simulink model "PID_Controller2_crazyfliemodel"  (R2016b)
settings: Solver=ode4  StartTime=0.0  StopTime=50  FixedStep=.01  RelTol=1e-5
InitFcn:
  | parameters;
values from neighbouring files (symbols this model uses):
  pwm = (we-4070.3)/0.2685    [parameters.m]
undefined symbols (not defined in the file or in its folder): delay1, quad
(part 1 of 2)
settings Model: Creator=corkep  LastModifiedBy=fmobini
settings SolverCC: AlgebraicLoopSolver=LineSearch
settings DataIOCC: LimitDataPoints=on  SaveFormat=Array  SignalLoggingSaveFormat=ModelDataLogs
settings OptimizationCC: BlockReduction=off  BooleanDataType=off  LifeSpan=inf
settings DebuggingCC: SaveWithParameterizedLinksMsg=none  UnderspecifiedInitializationDetection=Classic  MergeDetectMultiDrivingBlocksExec=none  SignalResolutionControl=TryResolveAllWithWarning  MultiTaskDSMMsg=warning  MultiTaskCondExecSysMsg=none  AllowSymbolicDim=off  StateNameClashWarn=warning  SFUnexpectedBacktrackingDiag=warning  SFNoUnconditionalDefaultTransitionDiag=warning  SFExecutionAtInitializationDiag=none
settings HardwareCC: ProdBitPerPointer=32  ProdBitPerSizeT=32  ProdBitPerPtrDiffT=32  ProdLargestAtomicFloat=None  ProdIntDivRoundTo=Undefined  ProdEndianess=Unspecified  ProdWordSize=32  ProdHWDeviceType=32-bit Generic  TargetBitPerPointer=64  TargetBitPerSizeT=64  TargetBitPerPtrDiffT=64  TargetLongLongMode=on  TargetIntDivRoundTo=Zero  TargetEndianess=LittleEndian  TargetWordSize=64  TargetHWDeviceType=MATLAB Host  ProdEqTarget=off
settings ModelReferenceCC: PropagateSignalLabelsOutOfModel=off
settings GRTTargetCC: TargetLangStandard=C89/C90 (ANSI)  GeneratePreprocessorConditionals=Disable all
settings ConfigComp: CovMetricSettings=dw  CovHtmlReporting=on  CovSaveCumulativeToWorkspaceVar=on  CovSaveSingleToWorkspaceVar=on  CovExternalEMLEnable=off

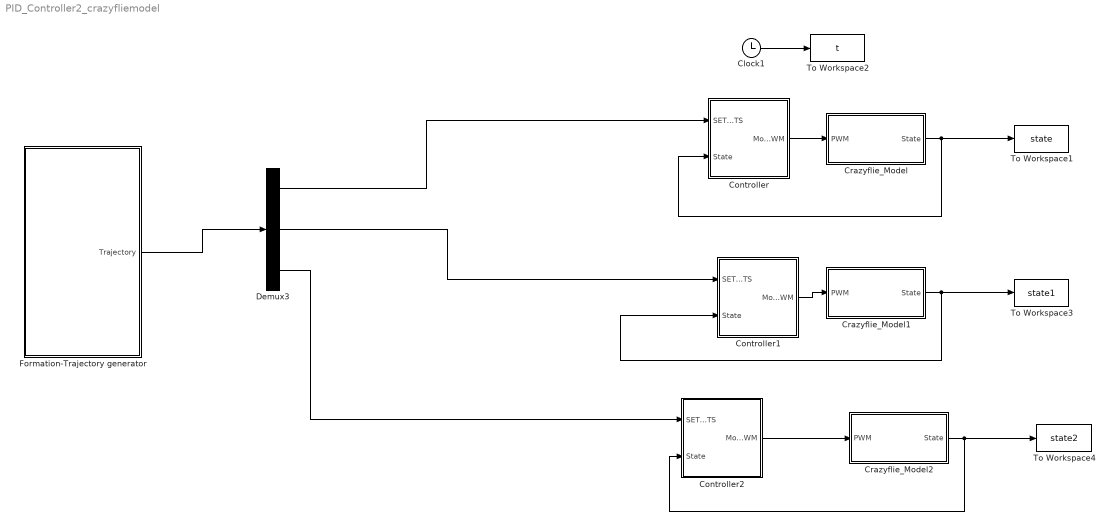
== system PID_Controller2_crazyfliemodel ==
  " Formation-Trajectory generator" : Subsystem
  Clock1 : Clock
  Controller : Subsystem  TreatAsAtomicUnit=on
  Controller1 : Subsystem  TreatAsAtomicUnit=on
  Controller2 : Subsystem  TreatAsAtomicUnit=on
  Crazyflie_Model : Subsystem
  Crazyflie_Model1 : Subsystem
  Crazyflie_Model2 : Subsystem
  Demux3 : Demux  Outputs=3
  To Workspace1 : ToWorkspace  VariableName=state  SampleTime=-1
  To Workspace2 : ToWorkspace  VariableName=t  SampleTime=-1
  To Workspace3 : ToWorkspace  VariableName=state1  SampleTime=-1
  To Workspace4 : ToWorkspace  VariableName=state2  SampleTime=-1
  wires:
  Clock1/1 -> To Workspace2/1
  Crazyflie_Model/1(State) -> To Workspace1/1, Controller/2(State)
  Controller/1(Motors_PWM) -> Crazyflie_Model/1(PWM)
  " Formation-Trajectory generator"/1(Trajectory) -> Demux3/1
  Demux3/1 -> Controller/1(SET-POINTS)
  Crazyflie_Model1/1(State) -> To Workspace3/1, Controller1/2(State)
  Controller1/1(Motors_PWM) -> Crazyflie_Model1/1(PWM)
  Demux3/2 -> Controller1/1(SET-POINTS)
  Crazyflie_Model2/1(State) -> To Workspace4/1, Controller2/2(State)
  Controller2/1(Motors_PWM) -> Crazyflie_Model2/1(PWM)
  Demux3/3 -> Controller2/1(SET-POINTS)

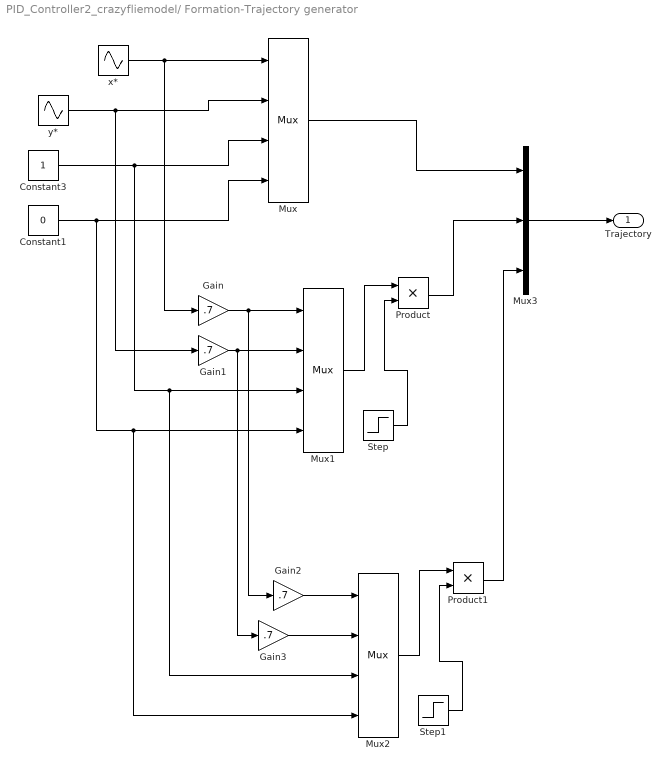
== system PID_Controller2_crazyfliemodel/ Formation-Trajectory generator ==
  Constant1 : Constant  Value=0
  Constant3 : Constant
  Gain{,1..3} (4 alike) : Gain  Gain=.7
  Mux : Mux
  Mux1 : Mux
  Mux2 : Mux
  Mux3 : Mux  Inputs=3
  Product : Product
  Product1 : Product
  Step : Step  Time=6  SampleTime=0
  Step1 : Step  Time=15  SampleTime=0
  x* : Sin  Amplitude=3  Frequency=2*pi*0.085
  y* : Sin  Amplitude=3  Frequency=2*pi*0.085  Phase=pi/2
  Trajectory : Outport
  wires:
  Constant3/1 -> Mux2/3, Mux1/3, Mux/3
  Constant1/1 -> Mux2/4, Mux1/4, Mux/4
  x*/1 -> Gain/1, Mux/1
  y*/1 -> Gain1/1, Mux/2
  Mux/1 -> Mux3/1
  Mux3/1 -> Trajectory/1
  Gain1/1 -> Gain3/1, Mux1/2
  Gain/1 -> Gain2/1, Mux1/1
  Gain2/1 -> Mux2/1
  Gain3/1 -> Mux2/2
  Product/1 -> Mux3/2
  Mux1/1 -> Product/1
  Step/1 -> Product/2
  Mux2/1 -> Product1/1
  Step1/1 -> Product1/2
  Product1/1 -> Mux3/3

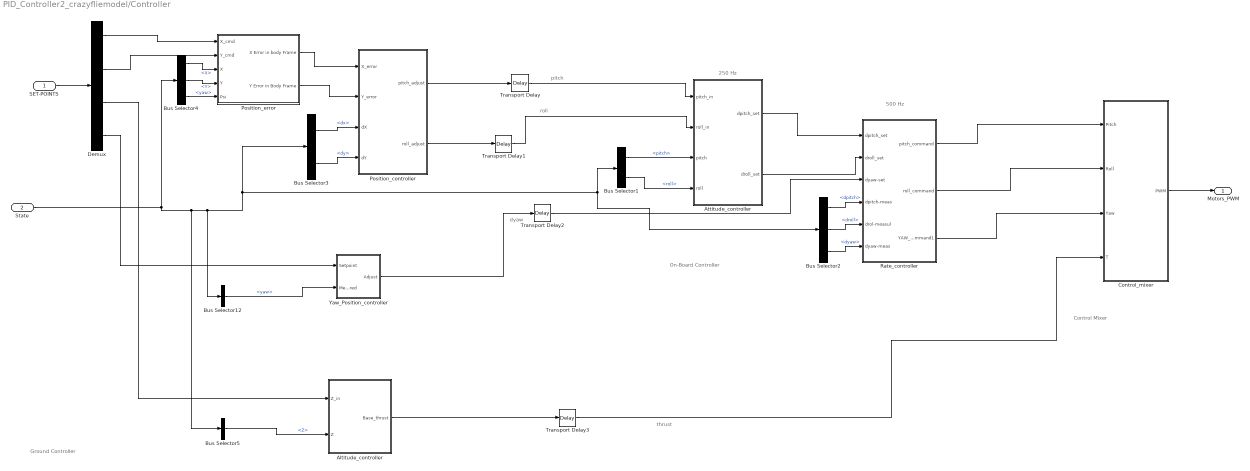
== system PID_Controller2_crazyfliemodel/Controller ==
  note: pitch
  note: Control Mixer
  note: On-Board Controller
  note: Ground Controller
  note: 250 Hz
  note: 500 Hz
  note: roll
  note: thrust
  note: dyaw
  SET-POINTS : Inport
  State : Inport  Port=2
  Altitude_controller : Subsystem
  Attitude_controller : Subsystem
  Bus Selector1 : BusSelector  OutputSignals=pitch,roll
  Bus Selector12 : BusSelector  OutputSignals=yaw
  Bus Selector2 : BusSelector  OutputSignals=dpitch,droll,dyaw
  Bus Selector3 : BusSelector  OutputSignals=dx,dy
  Bus Selector4 : BusSelector  OutputSignals=X,Y,yaw
  Bus Selector5 : BusSelector  OutputSignals=Z
  Control_mixer : Subsystem
  Demux : Demux
  Position_controller : Subsystem
  Position_error : Subsystem
  Rate_controller : Subsystem
  Transport Delay{,1..3} (4 alike) : TransportDelay  DelayTime=delay1
  Yaw_Position_controller : Subsystem
  Motors_PWM : Outport
  wires:
  Rate_controller/1(pitch_command) -> Control_mixer/1(Pitch)
  Rate_controller/2(roll_command) -> Control_mixer/2("Roll\t")
  Altitude_controller/1(Base_thrust) -> Transport Delay3/1
  Demux/3 -> Altitude_controller/1(Z_in)
  Bus Selector5/1 -> Altitude_controller/2(Z)  "<Z>"
  State/1 -> Bus Selector5/1, Bus Selector12/1, Bus Selector3/1, Bus Selector2/1, Bus Selector1/1, Bus Selector4/1
  Attitude_controller/1(dpitch_set) -> Rate_controller/1(dpitch_set)
  Attitude_controller/2(droll_set) -> Rate_controller/2(droll_set)
  Position_error/1(X Error in body Frame) -> Position_controller/1(X_error)
  Position_error/2(Y Error in Body Frame) -> Position_controller/2(Y_error)
  Position_controller/1(pitch_adjust) -> Transport Delay/1
  Bus Selector12/1 -> Yaw_Position_controller/2(Measured)  "<yaw>"
  Position_controller/2(roll_adjust) -> Transport Delay1/1
  Demux/1 -> Position_error/1(X_cmd)
  Demux/4 -> Yaw_Position_controller/1(Setpoint)
  Demux/2 -> Position_error/2(Y_cmd)
  SET-POINTS/1 -> Demux/1
  Yaw_Position_controller/1(Adjust) -> Transport Delay2/1
  Rate_controller/3(YAW_command1) -> Control_mixer/3(Yaw)
  Bus Selector1/1 -> Attitude_controller/3(pitch)  "<pitch>"
  Bus Selector1/2 -> Attitude_controller/4(roll)  "<roll>"
  Bus Selector2/1 -> Rate_controller/4(dpitch-meas)  "<dpitch>"
  Bus Selector2/2 -> Rate_controller/5(drol-measul)  "<droll>"
  Bus Selector2/3 -> Rate_controller/6(dyaw-meas)  "<dyaw>"
  Bus Selector3/1 -> Position_controller/3(dX)  "<dx>"
  Bus Selector3/2 -> Position_controller/4(dY)  "<dy>"
  Bus Selector4/1 -> Position_error/3(X)  "<X>"
  Bus Selector4/2 -> Position_error/4(Y)  "<Y>"
  Bus Selector4/3 -> Position_error/5(Psi)  "<yaw>"
  Control_mixer/1(PWM) -> Motors_PWM/1
  Transport Delay/1 -> Attitude_controller/1(pitch_in)
  Transport Delay1/1 -> Attitude_controller/2(roll_in)
  Transport Delay2/1 -> Rate_controller/3(dyaw-set)
  Transport Delay3/1 -> Control_mixer/4(T)

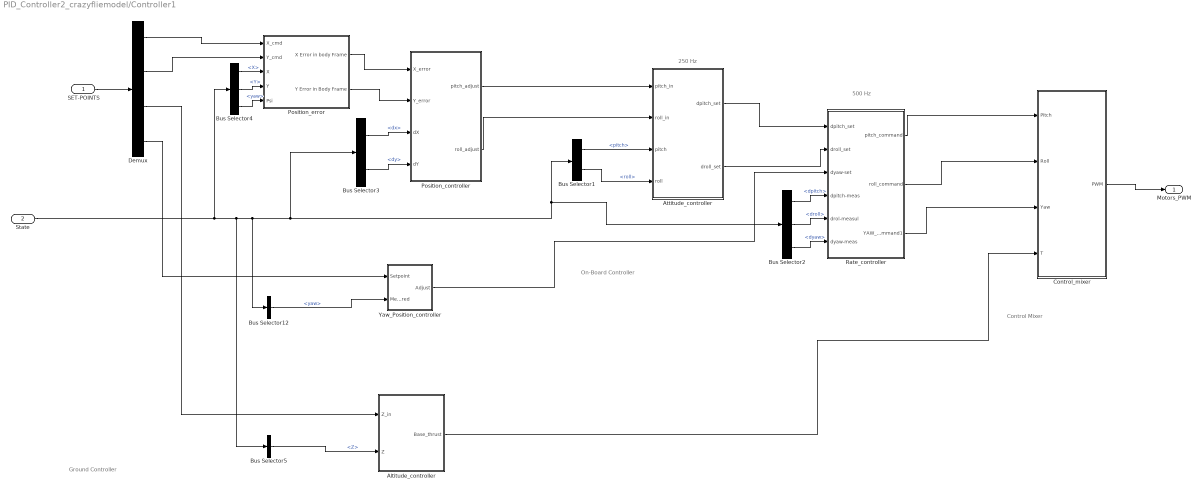
== system PID_Controller2_crazyfliemodel/Controller1 ==
  note: Control Mixer
  note: On-Board Controller
  note: Ground Controller
  note: 250 Hz
  note: 500 Hz
  SET-POINTS : Inport
  State : Inport  Port=2
  Altitude_controller : Subsystem
  Attitude_controller : Subsystem
  Bus Selector1 : BusSelector  OutputSignals=pitch,roll
  Bus Selector12 : BusSelector  OutputSignals=yaw
  Bus Selector2 : BusSelector  OutputSignals=dpitch,droll,dyaw
  Bus Selector3 : BusSelector  OutputSignals=dx,dy
  Bus Selector4 : BusSelector  OutputSignals=X,Y,yaw
  Bus Selector5 : BusSelector  OutputSignals=Z
  Control_mixer : Subsystem
  Demux : Demux
  Position_controller : Subsystem
  Position_error : Subsystem
  Rate_controller : Subsystem
  Yaw_Position_controller : Subsystem
  Motors_PWM : Outport
  wires:
  Control_mixer/1(PWM) -> Motors_PWM/1
  Rate_controller/1(pitch_command) -> Control_mixer/1(Pitch)
  Rate_controller/2(roll_command) -> Control_mixer/2("Roll\t")
  Altitude_controller/1(Base_thrust) -> Control_mixer/4(T)
  Demux/3 -> Altitude_controller/1(Z_in)
  Bus Selector5/1 -> Altitude_controller/2(Z)  "<Z>"
  State/1 -> Bus Selector4/1, Bus Selector5/1, Bus Selector12/1, Bus Selector3/1, Bus Selector2/1, Bus Selector1/1
  Attitude_controller/1(dpitch_set) -> Rate_controller/1(dpitch_set)
  Attitude_controller/2(droll_set) -> Rate_controller/2(droll_set)
  Position_error/1(X Error in body Frame) -> Position_controller/1(X_error)
  Position_error/2(Y Error in Body Frame) -> Position_controller/2(Y_error)
  Position_controller/1(pitch_adjust) -> Attitude_controller/1(pitch_in)
  Bus Selector12/1 -> Yaw_Position_controller/2(Measured)  "<yaw>"
  Position_controller/2(roll_adjust) -> Attitude_controller/2(roll_in)
  Demux/1 -> Position_error/1(X_cmd)
  Demux/4 -> Yaw_Position_controller/1(Setpoint)
  Demux/2 -> Position_error/2(Y_cmd)
  SET-POINTS/1 -> Demux/1
  Yaw_Position_controller/1(Adjust) -> Rate_controller/3(dyaw-set)
  Rate_controller/3(YAW_command1) -> Control_mixer/3(Yaw)
  Bus Selector1/1 -> Attitude_controller/3(pitch)  "<pitch>"
  Bus Selector1/2 -> Attitude_controller/4(roll)  "<roll>"
  Bus Selector2/1 -> Rate_controller/4(dpitch-meas)  "<dpitch>"
  Bus Selector2/2 -> Rate_controller/5(drol-measul)  "<droll>"
  Bus Selector2/3 -> Rate_controller/6(dyaw-meas)  "<dyaw>"
  Bus Selector3/1 -> Position_controller/3(dX)  "<dx>"
  Bus Selector3/2 -> Position_controller/4(dY)  "<dy>"
  Bus Selector4/1 -> Position_error/3(X)  "<X>"
  Bus Selector4/2 -> Position_error/4(Y)  "<Y>"
  Bus Selector4/3 -> Position_error/5(Psi)  "<yaw>"

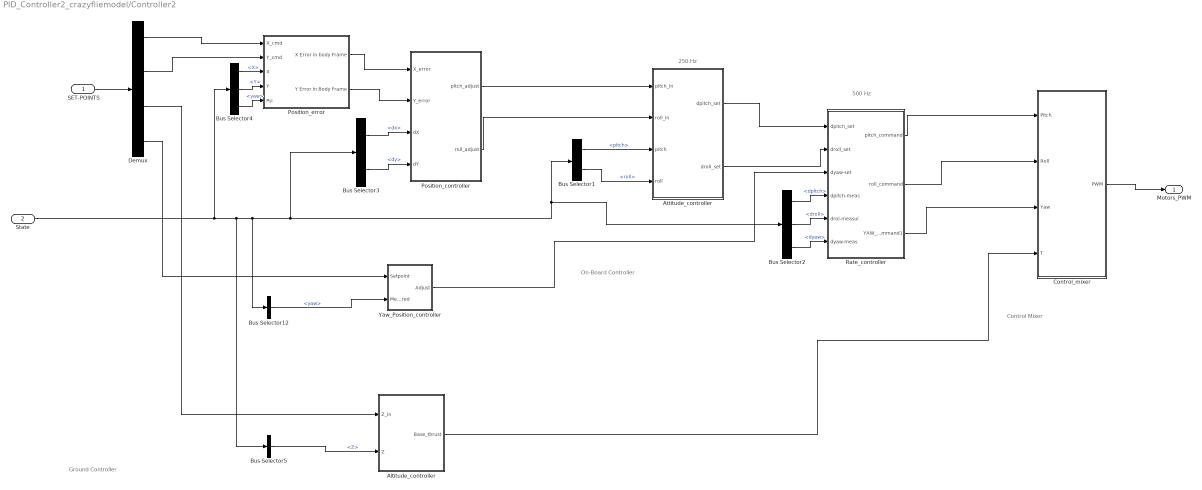
== system PID_Controller2_crazyfliemodel/Controller2 ==
  note: Control Mixer
  note: On-Board Controller
  note: Ground Controller
  note: 250 Hz
  note: 500 Hz
  SET-POINTS : Inport
  State : Inport  Port=2
  Altitude_controller : Subsystem
  Attitude_controller : Subsystem
  Bus Selector1 : BusSelector  OutputSignals=pitch,roll
  Bus Selector12 : BusSelector  OutputSignals=yaw
  Bus Selector2 : BusSelector  OutputSignals=dpitch,droll,dyaw
  Bus Selector3 : BusSelector  OutputSignals=dx,dy
  Bus Selector4 : BusSelector  OutputSignals=X,Y,yaw
  Bus Selector5 : BusSelector  OutputSignals=Z
  Control_mixer : Subsystem
  Demux : Demux
  Position_controller : Subsystem
  Position_error : Subsystem
  Rate_controller : Subsystem
  Yaw_Position_controller : Subsystem
  Motors_PWM : Outport
  wires:
  Control_mixer/1(PWM) -> Motors_PWM/1
  Rate_controller/1(pitch_command) -> Control_mixer/1(Pitch)
  Rate_controller/2(roll_command) -> Control_mixer/2("Roll\t")
  Altitude_controller/1(Base_thrust) -> Control_mixer/4(T)
  Demux/3 -> Altitude_controller/1(Z_in)
  Bus Selector5/1 -> Altitude_controller/2(Z)  "<Z>"
  State/1 -> Bus Selector4/1, Bus Selector5/1, Bus Selector12/1, Bus Selector3/1, Bus Selector2/1, Bus Selector1/1
  Attitude_controller/1(dpitch_set) -> Rate_controller/1(dpitch_set)
  Attitude_controller/2(droll_set) -> Rate_controller/2(droll_set)
  Position_error/1(X Error in body Frame) -> Position_controller/1(X_error)
  Position_error/2(Y Error in Body Frame) -> Position_controller/2(Y_error)
  Position_controller/1(pitch_adjust) -> Attitude_controller/1(pitch_in)
  Bus Selector12/1 -> Yaw_Position_controller/2(Measured)  "<yaw>"
  Position_controller/2(roll_adjust) -> Attitude_controller/2(roll_in)
  Demux/1 -> Position_error/1(X_cmd)
  Demux/4 -> Yaw_Position_controller/1(Setpoint)
  Demux/2 -> Position_error/2(Y_cmd)
  SET-POINTS/1 -> Demux/1
  Yaw_Position_controller/1(Adjust) -> Rate_controller/3(dyaw-set)
  Rate_controller/3(YAW_command1) -> Control_mixer/3(Yaw)
  Bus Selector1/1 -> Attitude_controller/3(pitch)  "<pitch>"
  Bus Selector1/2 -> Attitude_controller/4(roll)  "<roll>"
  Bus Selector2/1 -> Rate_controller/4(dpitch-meas)  "<dpitch>"
  Bus Selector2/2 -> Rate_controller/5(drol-measul)  "<droll>"
  Bus Selector2/3 -> Rate_controller/6(dyaw-meas)  "<dyaw>"
  Bus Selector3/1 -> Position_controller/3(dX)  "<dx>"
  Bus Selector3/2 -> Position_controller/4(dY)  "<dy>"
  Bus Selector4/1 -> Position_error/3(X)  "<X>"
  Bus Selector4/2 -> Position_error/4(Y)  "<Y>"
  Bus Selector4/3 -> Position_error/5(Psi)  "<yaw>"

== system PID_Controller2_crazyfliemodel/Crazyflie_Model ==
  PWM : Inport
  DYNAMICS MODEL : Subsystem
  Motor MODEL : Subsystem
  State : Outport
  wires:
  PWM/1 -> Motor MODEL/1(PWM)
  Motor MODEL/1(Thrust) -> DYNAMICS MODEL/1(THRUST)
  Motor MODEL/2(Moment) -> DYNAMICS MODEL/2(MOMENT)
  DYNAMICS MODEL/1(STATES) -> State/1

== system PID_Controller2_crazyfliemodel/Crazyflie_Model1 ==
  PWM : Inport
  DYNAMICS MODEL : Subsystem
  Motor MODEL : Subsystem
  State : Outport
  wires:
  PWM/1 -> Motor MODEL/1(PWM)
  Motor MODEL/1(Thrust) -> DYNAMICS MODEL/1(THRUST)
  Motor MODEL/2(Moment) -> DYNAMICS MODEL/2(MOMENT)
  DYNAMICS MODEL/1(STATES) -> State/1

== system PID_Controller2_crazyfliemodel/Crazyflie_Model2 ==
  PWM : Inport
  DYNAMICS MODEL : Subsystem
  Motor MODEL : Subsystem
  State : Outport
  wires:
  PWM/1 -> Motor MODEL/1(PWM)
  Motor MODEL/1(Thrust) -> DYNAMICS MODEL/1(THRUST)
  Motor MODEL/2(Moment) -> DYNAMICS MODEL/2(MOMENT)
  DYNAMICS MODEL/1(STATES) -> State/1

== system PID_Controller2_crazyfliemodel/Controller/Altitude_controller ==
  Z_in : Inport
  Z : Inport  Port=2
  "Min_thrust " : Constant  Value=pwm  SampleTime=0
  PID_Altitude : Subsystem
  Saturation : Saturate  UpperLimit=60000  LowerLimit=-20000
  Saturation1 : Saturate  UpperLimit=15000  LowerLimit=-20000
  Sum3 : Sum  Inputs=|++
  Base_thrust : Outport
  wires:
  Saturation/1 -> Base_thrust/1
  "Min_thrust "/1 -> Sum3/2
  Sum3/1 -> Saturation/1
  Z/1 -> PID_Altitude/2(Measured)
  Z_in/1 -> PID_Altitude/1(Setpoint)
  Saturation1/1 -> Sum3/1
  PID_Altitude/1(Adjust) -> Saturation1/1

== system PID_Controller2_crazyfliemodel/Controller/Attitude_controller ==
  pitch_in : Inport
  roll_in : Inport  Port=2
  pitch : Inport  Port=3
  roll : Inport  Port=4
  Gain1 : Gain  Gain=180/pi
  Gain3 : Gain  Gain=180/pi
  PID_pitch_Rate2 : Subsystem
  PID_roll_Rate1 : Subsystem
  dpitch_set : Outport
  droll_set : Outport  Port=2
  wires:
  roll_in/1 -> PID_roll_Rate1/1(Setpoint)
  roll/1 -> Gain1/1
  PID_roll_Rate1/1(Adjust) -> droll_set/1
  pitch_in/1 -> PID_pitch_Rate2/1(Setpoint)
  pitch/1 -> Gain3/1
  PID_pitch_Rate2/1(Adjust) -> dpitch_set/1
  Gain3/1 -> PID_pitch_Rate2/2(Measured)
  Gain1/1 -> PID_roll_Rate1/2(Measured)

== system PID_Controller2_crazyfliemodel/Controller/Control_mixer ==
  Pitch : Inport
  "Roll\t" : Inport  Port=2
  Yaw : Inport  Port=3
  T : Inport  Port=4
  Gain : Gain  Gain=0.5
  Gain1 : Gain  Gain=0.5
  Mux : Mux
  Sum1 : Sum  Inputs=|+-+  SaturateOnIntegerOverflow=on  InputSameDT=on  OutDataTypeStr=Inherit: Same as first input
  Sum{9..12} (4 alike) : Sum  Inputs=|++  SaturateOnIntegerOverflow=on  InputSameDT=on  OutDataTypeStr=Inherit: Same as first input
  Sum3 : Sum  Inputs=|++-  SaturateOnIntegerOverflow=on  InputSameDT=on  OutDataTypeStr=Inherit: Same as first input
  Sum5 : Sum  Inputs=|+-+  SaturateOnIntegerOverflow=on  InputSameDT=on  OutDataTypeStr=Inherit: Same as first input
  Sum7 : Sum  Inputs=|---  SaturateOnIntegerOverflow=on  InputSameDT=on  OutDataTypeStr=Inherit: Same as first input
  PWM : Outport
  wires:
  Sum3/1 -> Sum11/1
  Yaw/1 -> Sum5/3, Sum3/3, Sum7/3, Sum1/3
  T/1 -> Sum11/2, Sum12/2, Sum10/2, Sum9/2
  Sum5/1 -> Sum12/1
  Sum7/1 -> Sum9/1
  Sum1/1 -> Sum10/1
  "Roll\t"/1 -> Gain1/1
  Pitch/1 -> Gain/1
  Gain/1 -> Sum7/1, Sum1/1, Sum5/2, Sum3/2
  Gain1/1 -> Sum7/2, Sum1/2, Sum5/1, Sum3/1
  Sum9/1 -> Mux/1
  Sum10/1 -> Mux/2
  Sum11/1 -> Mux/3
  Sum12/1 -> Mux/4
  Mux/1 -> PWM/1

== system PID_Controller2_crazyfliemodel/Controller/Position_controller ==
  X_error : Inport
  Y_error : Inport  Port=2
  dX : Inport  Port=3
  dY : Inport  Port=4
  PID_pitch_Rate2 : Subsystem
  PID_roll_Rate3 : Subsystem
  Saturation : Saturate  UpperLimit=30  LowerLimit=-30
  Saturation1 : Saturate  UpperLimit=30  LowerLimit=-30
  Scope1 : Scope
  Scope2 : Scope
  pitch_adjust : Outport
  roll_adjust : Outport  Port=2
  wires:
  Saturation1/1 -> roll_adjust/1
  PID_roll_Rate3/1(Adjust) -> Saturation1/1
  Saturation/1 -> pitch_adjust/1, Scope1/1
  PID_pitch_Rate2/1(Adjust) -> Saturation/1, Scope2/1
  dX/1 -> PID_pitch_Rate2/2(Measured)
  X_error/1 -> PID_pitch_Rate2/1(Setpoint)
  dY/1 -> PID_roll_Rate3/2(Measured)
  Y_error/1 -> PID_roll_Rate3/1(Setpoint)

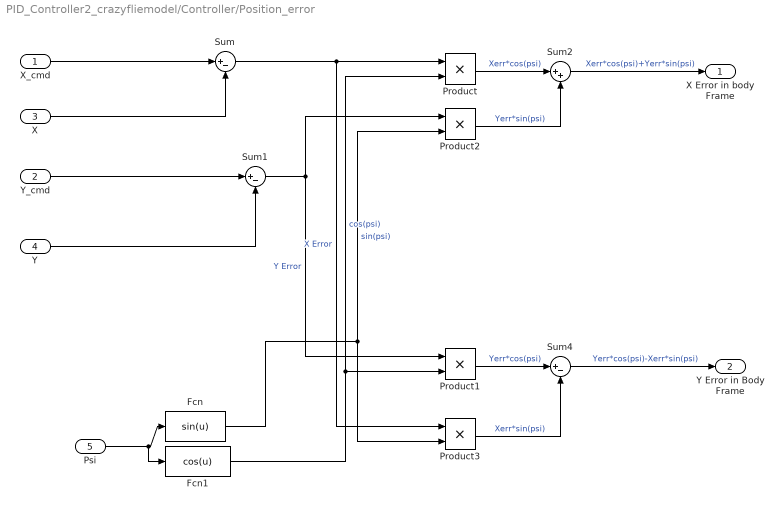
== system PID_Controller2_crazyfliemodel/Controller/Position_error ==
  X_cmd : Inport
  Y_cmd : Inport  Port=2
  X : Inport  Port=3
  Y : Inport  Port=4
  Psi : Inport  Port=5
  Fcn : Fcn  Expr=sin(u)
  Fcn1 : Fcn  Expr=cos(u)
  Product{,1..3} (4 alike) : Product
  Sum : Sum  Inputs=|+-
  Sum1 : Sum  Inputs=|+-
  Sum2 : Sum  Inputs=|++
  Sum4 : Sum  Inputs=|+-
  X Error in body Frame : Outport
  Y Error in Body Frame : Outport  Port=2
  wires:
  Sum4/1 -> Y Error in Body Frame/1  "Yerr*cos(psi)-Xerr*sin(psi)"
  Product3/1 -> Sum4/2  "Xerr*sin(psi)"
  Sum1/1 -> Product2/1, Product1/1  "Y Error"
  Fcn/1 -> Product3/2, Product2/2  "sin(psi)"
  Sum2/1 -> X Error in body Frame/1  "Xerr*cos(psi)+Yerr*sin(psi)"
  Y_cmd/1 -> Sum1/1
  X_cmd/1 -> Sum/1
  X/1 -> Sum/2
  Y/1 -> Sum1/2
  Sum/1 -> Product3/1, Product/1  "X Error"
  Fcn1/1 -> Product/2, Product1/2  "cos(psi)"
  Product/1 -> Sum2/1  "Xerr*cos(psi)"
  Product2/1 -> Sum2/2  "Yerr*sin(psi)"
  Product1/1 -> Sum4/1  "Yerr*cos(psi)"
  Psi/1 -> Fcn1/1, Fcn/1

== system PID_Controller2_crazyfliemodel/Controller/Rate_controller ==
  dpitch_set : Inport
  droll_set : Inport  Port=2
  dyaw-set : Inport  Port=3
  dpitch-meas : Inport  Port=4
  drol-measul : Inport  Port=5
  dyaw-meas : Inport  Port=6
  Gain1 : Gain  Gain=180/pi
  Gain4 : Gain  Gain=180/pi
  Gain7 : Gain  Gain=180/pi
  PID_Roll_Rate1 : Subsystem
  PID_Roll_Rate3 : Subsystem
  PID_YAW_Rate1 : Subsystem
  pitch_command : Outport
  roll_command : Outport  Port=2
  YAW_command1 : Outport  Port=3
  wires:
  dpitch_set/1 -> PID_Roll_Rate3/1(Setpoint)
  PID_Roll_Rate3/1(Adjust) -> pitch_command/1
  droll_set/1 -> PID_Roll_Rate1/1(Setpoint)
  drol-measul/1 -> Gain4/1
  PID_Roll_Rate1/1(Adjust) -> roll_command/1
  PID_YAW_Rate1/1(Adjust) -> YAW_command1/1
  dyaw-set/1 -> PID_YAW_Rate1/1(Setpoint)
  dyaw-meas/1 -> Gain7/1
  Gain7/1 -> PID_YAW_Rate1/2(Measured)
  Gain4/1 -> PID_Roll_Rate1/2(Measured)
  dpitch-meas/1 -> Gain1/1
  Gain1/1 -> PID_Roll_Rate3/2(Measured)

== system PID_Controller2_crazyfliemodel/Controller/Yaw_Position_controller ==
  Setpoint : Inport
  Measured : Inport  Port=2
  Gain6 : Gain  Gain=180/pi
  Kp : Gain  Gain=3  OutMin=[-200]  OutMax=[200]
  Saturation1 : Saturate  UpperLimit=200  LowerLimit=-200
  Sum6 : Sum  Inputs=+-|
  Adjust : Outport
  wires:
  Measured/1 -> Gain6/1  "measured"
  Setpoint/1 -> Sum6/1  "pid_desired"
  Kp/1 -> Saturation1/1
  Sum6/1 -> Kp/1  "pid_error"
  Gain6/1 -> Sum6/2
  Saturation1/1 -> Adjust/1

== system PID_Controller2_crazyfliemodel/Controller1/Altitude_controller ==
  Z_in : Inport
  Z : Inport  Port=2
  "Min_thrust " : Constant  Value=pwm  SampleTime=0
  PID_Altitude : Subsystem
  Saturation : Saturate  UpperLimit=60000  LowerLimit=-20000
  Saturation1 : Saturate  UpperLimit=15000  LowerLimit=-20000
  Sum3 : Sum  Inputs=|++
  Base_thrust : Outport
  wires:
  Saturation/1 -> Base_thrust/1
  "Min_thrust "/1 -> Sum3/2
  Sum3/1 -> Saturation/1
  Z/1 -> PID_Altitude/2(Measured)
  Z_in/1 -> PID_Altitude/1(Setpoint)
  Saturation1/1 -> Sum3/1
  PID_Altitude/1(Adjust) -> Saturation1/1

== system PID_Controller2_crazyfliemodel/Controller1/Attitude_controller ==
  pitch_in : Inport
  roll_in : Inport  Port=2
  pitch : Inport  Port=3
  roll : Inport  Port=4
  Gain1 : Gain  Gain=180/pi
  Gain3 : Gain  Gain=180/pi
  PID_Roll_Rate1 : Subsystem
  PID_Roll_Rate2 : Subsystem
  dpitch_set : Outport
  droll_set : Outport  Port=2
  wires:
  roll_in/1 -> PID_Roll_Rate1/1(Setpoint)
  roll/1 -> Gain1/1
  PID_Roll_Rate1/1(Adjust) -> droll_set/1
  pitch_in/1 -> PID_Roll_Rate2/1(Setpoint)
  pitch/1 -> Gain3/1
  PID_Roll_Rate2/1(Adjust) -> dpitch_set/1
  Gain3/1 -> PID_Roll_Rate2/2(Measured)
  Gain1/1 -> PID_Roll_Rate1/2(Measured)

== system PID_Controller2_crazyfliemodel/Controller1/Control_mixer ==
  Pitch : Inport
  "Roll\t" : Inport  Port=2
  Yaw : Inport  Port=3
  T : Inport  Port=4
  Configuration_X1 : Subsystem
  Mux1 : Mux
  PWM : Outport
  wires:
  Pitch/1 -> Configuration_X1/1(Pitch)
  Configuration_X1/3(W3) -> Mux1/3
  Configuration_X1/4(W4) -> Mux1/4
  T/1 -> Configuration_X1/4(Tau)
  Yaw/1 -> Configuration_X1/3(Yaw)
  "Roll\t"/1 -> Configuration_X1/2(Roll)
  Configuration_X1/2(W2) -> Mux1/2
  Configuration_X1/1(W1) -> Mux1/1
  Mux1/1 -> PWM/1

== system PID_Controller2_crazyfliemodel/Controller1/Position_controller ==
  X_error : Inport
  Y_error : Inport  Port=2
  dX : Inport  Port=3
  dY : Inport  Port=4
  PID_Roll_Rate2 : Subsystem
  PID_Roll_Rate3 : Subsystem
  PID_X2 : Subsystem
  PID_Y2 : Subsystem
  Saturation : Saturate  UpperLimit=30  LowerLimit=-30
  Saturation1 : Saturate  UpperLimit=30  LowerLimit=-30
  Scope1 : Scope
  Scope2 : Scope
  pitch_adjust : Outport
  roll_adjust : Outport  Port=2
  wires:
  Saturation1/1 -> roll_adjust/1
  PID_Roll_Rate3/1(Adjust) -> Saturation1/1
  Saturation/1 -> pitch_adjust/1, Scope1/1
  PID_Roll_Rate2/1(Adjust) -> Saturation/1, Scope2/1
  dX/1 -> PID_Roll_Rate2/2(Measured)
  X_error/1 -> PID_Roll_Rate2/1(Setpoint)
  dY/1 -> PID_Roll_Rate3/2(Measured)
  Y_error/1 -> PID_Roll_Rate3/1(Setpoint)

== system PID_Controller2_crazyfliemodel/Controller1/Position_error ==
  X_cmd : Inport
  Y_cmd : Inport  Port=2
  X : Inport  Port=3
  Y : Inport  Port=4
  Psi : Inport  Port=5
  Fcn : Fcn  Expr=sin(u)
  Fcn1 : Fcn  Expr=cos(u)
  Product{,1..3} (4 alike) : Product
  Sum : Sum  Inputs=|+-
  Sum1 : Sum  Inputs=|+-
  Sum2 : Sum  Inputs=|++
  Sum4 : Sum  Inputs=|+-
  X Error in body Frame : Outport
  Y Error in Body Frame : Outport  Port=2
  wires:
  Sum4/1 -> Y Error in Body Frame/1  "Yerr*cos(psi)-Xerr*sin(psi)"
  Product3/1 -> Sum4/2  "Xerr*sin(psi)"
  Sum1/1 -> Product2/1, Product1/1  "Y Error"
  Fcn/1 -> Product3/2, Product2/2  "sin(psi)"
  Sum2/1 -> X Error in body Frame/1  "Xerr*cos(psi)+Yerr*sin(psi)"
  Y_cmd/1 -> Sum1/1
  X_cmd/1 -> Sum/1
  X/1 -> Sum/2
  Y/1 -> Sum1/2
  Sum/1 -> Product3/1, Product/1  "X Error"
  Fcn1/1 -> Product/2, Product1/2  "cos(psi)"
  Product/1 -> Sum2/1  "Xerr*cos(psi)"
  Product2/1 -> Sum2/2  "Yerr*sin(psi)"
  Product1/1 -> Sum4/1  "Yerr*cos(psi)"
  Psi/1 -> Fcn1/1, Fcn/1

== system PID_Controller2_crazyfliemodel/Controller1/Rate_controller ==
  dpitch_set : Inport
  droll_set : Inport  Port=2
  dyaw-set : Inport  Port=3
  dpitch-meas : Inport  Port=4
  drol-measul : Inport  Port=5
  dyaw-meas : Inport  Port=6
  Gain1 : Gain  Gain=180/pi
  Gain4 : Gain  Gain=180/pi
  Gain7 : Gain  Gain=180/pi
  PID_Roll_Rate1 : Subsystem
  PID_Roll_Rate3 : Subsystem
  PID_YAW_Rate1 : Subsystem
  pitch_command : Outport
  roll_command : Outport  Port=2
  YAW_command1 : Outport  Port=3
  wires:
  dpitch_set/1 -> PID_Roll_Rate3/1(Setpoint)
  PID_Roll_Rate3/1(Adjust) -> pitch_command/1
  droll_set/1 -> PID_Roll_Rate1/1(Setpoint)
  drol-measul/1 -> Gain4/1
  PID_Roll_Rate1/1(Adjust) -> roll_command/1
  PID_YAW_Rate1/1(Adjust) -> YAW_command1/1
  dyaw-set/1 -> PID_YAW_Rate1/1(Setpoint)
  dyaw-meas/1 -> Gain7/1
  Gain7/1 -> PID_YAW_Rate1/2(Measured)
  Gain4/1 -> PID_Roll_Rate1/2(Measured)
  dpitch-meas/1 -> Gain1/1
  Gain1/1 -> PID_Roll_Rate3/2(Measured)

== system PID_Controller2_crazyfliemodel/Controller1/Yaw_Position_controller ==
  Setpoint : Inport
  Measured : Inport  Port=2
  Gain6 : Gain  Gain=180/pi
  Kp : Gain  Gain=3  OutMin=[-200]  OutMax=[200]
  Saturation1 : Saturate  UpperLimit=200  LowerLimit=-200
  Sum6 : Sum  Inputs=+-|
  Adjust : Outport
  wires:
  Measured/1 -> Gain6/1  "measured"
  Setpoint/1 -> Sum6/1  "pid_desired"
  Kp/1 -> Saturation1/1
  Sum6/1 -> Kp/1  "pid_error"
  Gain6/1 -> Sum6/2
  Saturation1/1 -> Adjust/1

== system PID_Controller2_crazyfliemodel/Controller2/Altitude_controller ==
  Z_in : Inport
  Z : Inport  Port=2
  "Min_thrust " : Constant  Value=pwm  SampleTime=0
  PID_Altitude : Subsystem
  Saturation : Saturate  UpperLimit=60000  LowerLimit=-20000
  Saturation1 : Saturate  UpperLimit=15000  LowerLimit=-20000
  Sum3 : Sum  Inputs=|++
  Base_thrust : Outport
  wires:
  Saturation/1 -> Base_thrust/1
  "Min_thrust "/1 -> Sum3/2
  Sum3/1 -> Saturation/1
  Z/1 -> PID_Altitude/2(Measured)
  Z_in/1 -> PID_Altitude/1(Setpoint)
  Saturation1/1 -> Sum3/1
  PID_Altitude/1(Adjust) -> Saturation1/1

== system PID_Controller2_crazyfliemodel/Controller2/Attitude_controller ==
  pitch_in : Inport
  roll_in : Inport  Port=2
  pitch : Inport  Port=3
  roll : Inport  Port=4
  Gain1 : Gain  Gain=180/pi
  Gain3 : Gain  Gain=180/pi
  PID_Roll_Rate1 : Subsystem
  PID_Roll_Rate2 : Subsystem
  dpitch_set : Outport
  droll_set : Outport  Port=2
  wires:
  roll_in/1 -> PID_Roll_Rate1/1(Setpoint)
  roll/1 -> Gain1/1
  PID_Roll_Rate1/1(Adjust) -> droll_set/1
  pitch_in/1 -> PID_Roll_Rate2/1(Setpoint)
  pitch/1 -> Gain3/1
  PID_Roll_Rate2/1(Adjust) -> dpitch_set/1
  Gain3/1 -> PID_Roll_Rate2/2(Measured)
  Gain1/1 -> PID_Roll_Rate1/2(Measured)

== system PID_Controller2_crazyfliemodel/Controller2/Control_mixer ==
  Pitch : Inport
  "Roll\t" : Inport  Port=2
  Yaw : Inport  Port=3
  T : Inport  Port=4
  Configuration_X1 : Subsystem
  Mux1 : Mux
  PWM : Outport
  wires:
  Pitch/1 -> Configuration_X1/1(Pitch)
  Configuration_X1/3(W3) -> Mux1/3
  Configuration_X1/4(W4) -> Mux1/4
  T/1 -> Configuration_X1/4(Tau)
  Yaw/1 -> Configuration_X1/3(Yaw)
  "Roll\t"/1 -> Configuration_X1/2(Roll)
  Configuration_X1/2(W2) -> Mux1/2
  Configuration_X1/1(W1) -> Mux1/1
  Mux1/1 -> PWM/1

== system PID_Controller2_crazyfliemodel/Controller2/Position_controller ==
  X_error : Inport
  Y_error : Inport  Port=2
  dX : Inport  Port=3
  dY : Inport  Port=4
  PID_Roll_Rate2 : Subsystem
  PID_Roll_Rate3 : Subsystem
  PID_X2 : Subsystem
  PID_Y2 : Subsystem
  Saturation : Saturate  UpperLimit=30  LowerLimit=-30
  Saturation1 : Saturate  UpperLimit=30  LowerLimit=-30
  Scope1 : Scope
  Scope2 : Scope
  pitch_adjust : Outport
  roll_adjust : Outport  Port=2
  wires:
  Saturation1/1 -> roll_adjust/1
  PID_Roll_Rate3/1(Adjust) -> Saturation1/1
  Saturation/1 -> pitch_adjust/1, Scope1/1
  PID_Roll_Rate2/1(Adjust) -> Saturation/1, Scope2/1
  dX/1 -> PID_Roll_Rate2/2(Measured)
  X_error/1 -> PID_Roll_Rate2/1(Setpoint)
  dY/1 -> PID_Roll_Rate3/2(Measured)
  Y_error/1 -> PID_Roll_Rate3/1(Setpoint)

== system PID_Controller2_crazyfliemodel/Controller2/Position_error ==
  X_cmd : Inport
  Y_cmd : Inport  Port=2
  X : Inport  Port=3
  Y : Inport  Port=4
  Psi : Inport  Port=5
  Fcn : Fcn  Expr=sin(u)
  Fcn1 : Fcn  Expr=cos(u)
  Product{,1..3} (4 alike) : Product
  Sum : Sum  Inputs=|+-
  Sum1 : Sum  Inputs=|+-
  Sum2 : Sum  Inputs=|++
  Sum4 : Sum  Inputs=|+-
  X Error in body Frame : Outport
  Y Error in Body Frame : Outport  Port=2
  wires:
  Sum4/1 -> Y Error in Body Frame/1  "Yerr*cos(psi)-Xerr*sin(psi)"
  Product3/1 -> Sum4/2  "Xerr*sin(psi)"
  Sum1/1 -> Product2/1, Product1/1  "Y Error"
  Fcn/1 -> Product3/2, Product2/2  "sin(psi)"
  Sum2/1 -> X Error in body Frame/1  "Xerr*cos(psi)+Yerr*sin(psi)"
  Y_cmd/1 -> Sum1/1
  X_cmd/1 -> Sum/1
  X/1 -> Sum/2
  Y/1 -> Sum1/2
  Sum/1 -> Product3/1, Product/1  "X Error"
  Fcn1/1 -> Product/2, Product1/2  "cos(psi)"
  Product/1 -> Sum2/1  "Xerr*cos(psi)"
  Product2/1 -> Sum2/2  "Yerr*sin(psi)"
  Product1/1 -> Sum4/1  "Yerr*cos(psi)"
  Psi/1 -> Fcn1/1, Fcn/1

== system PID_Controller2_crazyfliemodel/Controller2/Rate_controller ==
  dpitch_set : Inport
  droll_set : Inport  Port=2
  dyaw-set : Inport  Port=3
  dpitch-meas : Inport  Port=4
  drol-measul : Inport  Port=5
  dyaw-meas : Inport  Port=6
  Gain1 : Gain  Gain=180/pi
  Gain4 : Gain  Gain=180/pi
  Gain7 : Gain  Gain=180/pi
  PID_Roll_Rate1 : Subsystem
  PID_Roll_Rate3 : Subsystem
  PID_YAW_Rate1 : Subsystem
  pitch_command : Outport
  roll_command : Outport  Port=2
  YAW_command1 : Outport  Port=3
  wires:
  dpitch_set/1 -> PID_Roll_Rate3/1(Setpoint)
  PID_Roll_Rate3/1(Adjust) -> pitch_command/1
  droll_set/1 -> PID_Roll_Rate1/1(Setpoint)
  drol-measul/1 -> Gain4/1
  PID_Roll_Rate1/1(Adjust) -> roll_command/1
  PID_YAW_Rate1/1(Adjust) -> YAW_command1/1
  dyaw-set/1 -> PID_YAW_Rate1/1(Setpoint)
  dyaw-meas/1 -> Gain7/1
  Gain7/1 -> PID_YAW_Rate1/2(Measured)
  Gain4/1 -> PID_Roll_Rate1/2(Measured)
  dpitch-meas/1 -> Gain1/1
  Gain1/1 -> PID_Roll_Rate3/2(Measured)

== system PID_Controller2_crazyfliemodel/Controller2/Yaw_Position_controller ==
  Setpoint : Inport
  Measured : Inport  Port=2
  Gain6 : Gain  Gain=180/pi
  Kp : Gain  Gain=3  OutMin=[-200]  OutMax=[200]
  Saturation1 : Saturate  UpperLimit=200  LowerLimit=-200
  Sum6 : Sum  Inputs=+-|
  Adjust : Outport
  wires:
  Measured/1 -> Gain6/1  "measured"
  Setpoint/1 -> Sum6/1  "pid_desired"
  Kp/1 -> Saturation1/1
  Sum6/1 -> Kp/1  "pid_error"
  Gain6/1 -> Sum6/2
  Saturation1/1 -> Adjust/1

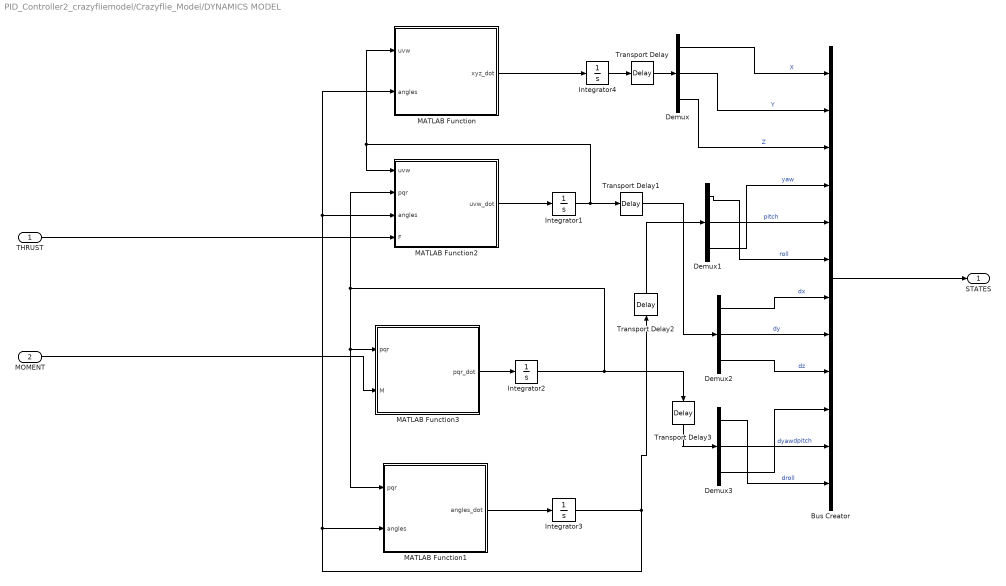
== system PID_Controller2_crazyfliemodel/Crazyflie_Model/DYNAMICS MODEL ==
  THRUST : Inport
  MOMENT : Inport  Port=2
  Bus Creator : BusCreator  Inputs=12
  Demux{,1..3} (4 alike) : Demux  Outputs=3
  Integrator1 : Integrator
  Integrator2 : Integrator
  Integrator3 : Integrator
  Integrator4 : Integrator  InitialCondition=[0;0;0]
  MATLAB Function : MATLAB Function  TreatAsAtomicUnit=on
  MATLAB Function1 : MATLAB Function  TreatAsAtomicUnit=on
  MATLAB Function2 : MATLAB Function  TreatAsAtomicUnit=on
  MATLAB Function3 : MATLAB Function  TreatAsAtomicUnit=on
  Transport Delay{,1..3} (4 alike) : TransportDelay  DelayTime=delay1
  STATES : Outport
  wires:
  MATLAB Function/1(xyz_dot) -> Integrator4/1
  MATLAB Function2/1(uvw_dot) -> Integrator1/1
  MATLAB Function1/1(angles_dot) -> Integrator3/1
  MATLAB Function3/1(pqr_dot) -> Integrator2/1
  Demux/2 -> Bus Creator/2  "Y"
  Demux3/2 -> Bus Creator/11  "dpitch"
  Demux/1 -> Bus Creator/1  "X"
  Demux3/1 -> Bus Creator/12  "droll"
  Integrator3/1 -> Transport Delay2/1, MATLAB Function/2(angles), MATLAB Function2/3(angles), MATLAB Function1/2(angles)
  Demux1/3 -> Bus Creator/4  "yaw"
  Demux2/1 -> Bus Creator/7  "dx"
  Demux2/3 -> Bus Creator/9  "dz"
  Integrator1/1 -> Transport Delay1/1, MATLAB Function/1(uvw), MATLAB Function2/1(uvw)
  Demux3/3 -> Bus Creator/10  "dyaw"
  Demux/3 -> Bus Creator/3  "Z"
  Integrator4/1 -> Transport Delay/1
  Demux1/2 -> Bus Creator/5  "pitch"
  Demux1/1 -> Bus Creator/6  "roll"
  Demux2/2 -> Bus Creator/8  "dy"
  Integrator2/1 -> Transport Delay3/1, MATLAB Function2/2(pqr), MATLAB Function1/1(pqr), MATLAB Function3/1(pqr)
  THRUST/1 -> MATLAB Function2/4(F)
  MOMENT/1 -> MATLAB Function3/2(M)
  Bus Creator/1 -> STATES/1
  Transport Delay/1 -> Demux/1
  Transport Delay1/1 -> Demux2/1
  Transport Delay2/1 -> Demux1/1
  Transport Delay3/1 -> Demux3/1

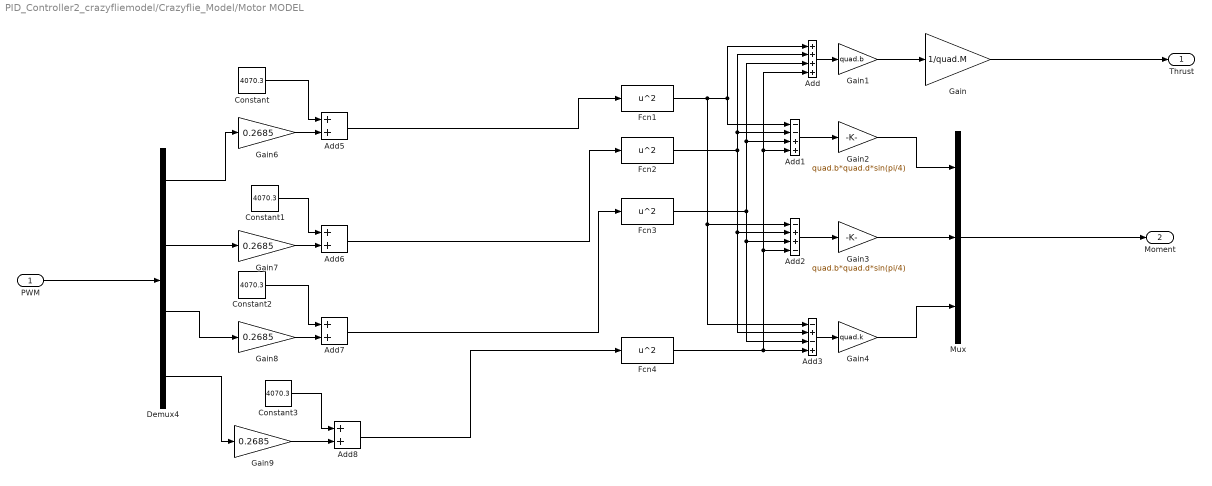
== system PID_Controller2_crazyfliemodel/Crazyflie_Model/Motor MODEL ==
  PWM : Inport
  Add : Sum  Inputs=++++
  Add1 : Sum  Inputs=--++
  Add2 : Sum  Inputs=-++-
  Add3 : Sum  Inputs=-+-+
  Add{5..8} (4 alike) : Sum
  Constant{,1..3} (4 alike) : Constant  Value=4070.3
  Demux4 : Demux
  Fcn{1..4} (4 alike) : Fcn  Expr=u^2
  Gain : Gain  Gain=1/quad.M
  Gain1 : Gain  Gain=quad.b
  Gain2 : Gain  Gain=quad.b*quad.d*sin(pi/4)
  Gain3 : Gain  Gain=quad.b*quad.d*sin(pi/4)
  Gain4 : Gain  Gain=quad.k
  Gain{6..9} (4 alike) : Gain  Gain=0.2685
  Mux : Mux  Inputs=3
  Thrust : Outport
  Moment : Outport  Port=2
  wires:
  Fcn1/1 -> Add/1, Add1/1, Add2/1, Add3/1
  Add1/1 -> Gain2/1
  Add6/1 -> Fcn2/1
  Fcn3/1 -> Add1/3, Add/3, Add2/3, Add3/3
  Add/1 -> Gain1/1
  Gain2/1 -> Mux/1
  Gain4/1 -> Mux/3
  Fcn2/1 -> Add2/2, Add3/2, Add1/2, Add/2
  Add3/1 -> Gain4/1
  Add2/1 -> Gain3/1
  Add7/1 -> Fcn3/1
  Mux/1 -> Moment/1
  Gain1/1 -> Gain/1
  Add5/1 -> Fcn1/1
  Gain3/1 -> Mux/2
  Add8/1 -> Fcn4/1
  Fcn4/1 -> Add/4, Add1/4, Add2/4, Add3/4
  Gain/1 -> Thrust/1
  Constant2/1 -> Add7/1
  PWM/1 -> Demux4/1
  Constant/1 -> Add5/1
  Gain8/1 -> Add7/2
  Demux4/3 -> Gain8/1
  Gain9/1 -> Add8/2
  Constant1/1 -> Add6/1
  Demux4/2 -> Gain7/1
  Demux4/1 -> Gain6/1
  Constant3/1 -> Add8/1
  Demux4/4 -> Gain9/1
  Gain7/1 -> Add6/2
  Gain6/1 -> Add5/2

== system PID_Controller2_crazyfliemodel/Crazyflie_Model1/DYNAMICS MODEL ==
  THRUST : Inport
  MOMENT : Inport  Port=2
  Bus Creator : BusCreator  Inputs=12
  Demux{,1..3} (4 alike) : Demux  Outputs=3
  Integrator1 : Integrator
  Integrator2 : Integrator
  Integrator3 : Integrator
  Integrator4 : Integrator  InitialCondition=[0;0;0]
  MATLAB Function : MATLAB Function  TreatAsAtomicUnit=on
  MATLAB Function1 : MATLAB Function  TreatAsAtomicUnit=on
  MATLAB Function2 : MATLAB Function  TreatAsAtomicUnit=on
  MATLAB Function3 : MATLAB Function  TreatAsAtomicUnit=on
  STATES : Outport
  wires:
  Bus Creator/1 -> STATES/1
  MATLAB Function/1(xyz_dot) -> Integrator4/1
  MATLAB Function2/1(uvw_dot) -> Integrator1/1
  MATLAB Function1/1(angles_dot) -> Integrator3/1
  MATLAB Function3/1(pqr_dot) -> Integrator2/1
  Demux/2 -> Bus Creator/2  "Y"
  Demux3/2 -> Bus Creator/11  "dpitch"
  Demux/1 -> Bus Creator/1  "X"
  Demux3/1 -> Bus Creator/12  "droll"
  Integrator3/1 -> Demux1/1, MATLAB Function/2(angles), MATLAB Function2/3(angles), MATLAB Function1/2(angles)
  Demux1/3 -> Bus Creator/4  "yaw"
  Demux2/1 -> Bus Creator/7  "dx"
  Demux2/3 -> Bus Creator/9  "dz"
  Integrator1/1 -> Demux2/1, MATLAB Function/1(uvw), MATLAB Function2/1(uvw)
  Demux3/3 -> Bus Creator/10  "dyaw"
  Demux/3 -> Bus Creator/3  "Z"
  Integrator4/1 -> Demux/1
  Demux1/2 -> Bus Creator/5  "pitch"
  Demux1/1 -> Bus Creator/6  "roll"
  Demux2/2 -> Bus Creator/8  "dy"
  Integrator2/1 -> Demux3/1, MATLAB Function2/2(pqr), MATLAB Function1/1(pqr), MATLAB Function3/1(pqr)
  THRUST/1 -> MATLAB Function2/4(F)
  MOMENT/1 -> MATLAB Function3/2(M)

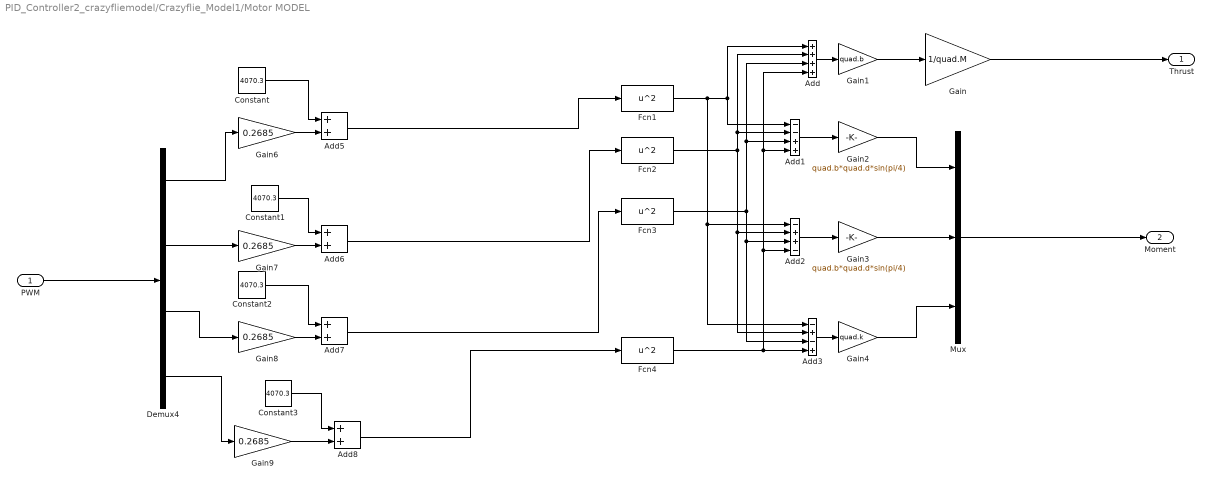
== system PID_Controller2_crazyfliemodel/Crazyflie_Model1/Motor MODEL ==
  PWM : Inport
  Add : Sum  Inputs=++++
  Add1 : Sum  Inputs=--++
  Add2 : Sum  Inputs=-++-
  Add3 : Sum  Inputs=-+-+
  Add{5..8} (4 alike) : Sum
  Constant{,1..3} (4 alike) : Constant  Value=4070.3
  Demux4 : Demux
  Fcn{1..4} (4 alike) : Fcn  Expr=u^2
  Gain : Gain  Gain=1/quad.M
  Gain1 : Gain  Gain=quad.b
  Gain2 : Gain  Gain=quad.b*quad.d*sin(pi/4)
  Gain3 : Gain  Gain=quad.b*quad.d*sin(pi/4)
  Gain4 : Gain  Gain=quad.k
  Gain{6..9} (4 alike) : Gain  Gain=0.2685
  Mux : Mux  Inputs=3
  Thrust : Outport
  Moment : Outport  Port=2
  wires:
  Fcn1/1 -> Add/1, Add1/1, Add2/1, Add3/1
  Add1/1 -> Gain2/1
  Add6/1 -> Fcn2/1
  Fcn3/1 -> Add1/3, Add/3, Add2/3, Add3/3
  Add/1 -> Gain1/1
  Gain2/1 -> Mux/1
  Gain4/1 -> Mux/3
  Fcn2/1 -> Add2/2, Add3/2, Add1/2, Add/2
  Add3/1 -> Gain4/1
  Add2/1 -> Gain3/1
  Add7/1 -> Fcn3/1
  Mux/1 -> Moment/1
  Gain1/1 -> Gain/1
  Add5/1 -> Fcn1/1
  Gain3/1 -> Mux/2
  Add8/1 -> Fcn4/1
  Fcn4/1 -> Add/4, Add1/4, Add2/4, Add3/4
  Gain/1 -> Thrust/1
  Constant2/1 -> Add7/1
  PWM/1 -> Demux4/1
  Constant/1 -> Add5/1
  Gain8/1 -> Add7/2
  Demux4/3 -> Gain8/1
  Gain9/1 -> Add8/2
  Constant1/1 -> Add6/1
  Demux4/2 -> Gain7/1
  Demux4/1 -> Gain6/1
  Constant3/1 -> Add8/1
  Demux4/4 -> Gain9/1
  Gain7/1 -> Add6/2
  Gain6/1 -> Add5/2

== system PID_Controller2_crazyfliemodel/Crazyflie_Model2/DYNAMICS MODEL ==
  THRUST : Inport
  MOMENT : Inport  Port=2
  Bus Creator : BusCreator  Inputs=12
  Demux{,1..3} (4 alike) : Demux  Outputs=3
  Integrator1 : Integrator
  Integrator2 : Integrator
  Integrator3 : Integrator
  Integrator4 : Integrator  InitialCondition=[0;0;0]
  MATLAB Function : MATLAB Function  TreatAsAtomicUnit=on
  MATLAB Function1 : MATLAB Function  TreatAsAtomicUnit=on
  MATLAB Function2 : MATLAB Function  TreatAsAtomicUnit=on
  MATLAB Function3 : MATLAB Function  TreatAsAtomicUnit=on
  STATES : Outport
  wires:
  Bus Creator/1 -> STATES/1
  MATLAB Function/1(xyz_dot) -> Integrator4/1
  MATLAB Function2/1(uvw_dot) -> Integrator1/1
  MATLAB Function1/1(angles_dot) -> Integrator3/1
  MATLAB Function3/1(pqr_dot) -> Integrator2/1
  Demux/2 -> Bus Creator/2  "Y"
  Demux3/2 -> Bus Creator/11  "dpitch"
  Demux/1 -> Bus Creator/1  "X"
  Demux3/1 -> Bus Creator/12  "droll"
  Integrator3/1 -> Demux1/1, MATLAB Function/2(angles), MATLAB Function2/3(angles), MATLAB Function1/2(angles)
  Demux1/3 -> Bus Creator/4  "yaw"
  Demux2/1 -> Bus Creator/7  "dx"
  Demux2/3 -> Bus Creator/9  "dz"
  Integrator1/1 -> Demux2/1, MATLAB Function/1(uvw), MATLAB Function2/1(uvw)
  Demux3/3 -> Bus Creator/10  "dyaw"
  Demux/3 -> Bus Creator/3  "Z"
  Integrator4/1 -> Demux/1
  Demux1/2 -> Bus Creator/5  "pitch"
  Demux1/1 -> Bus Creator/6  "roll"
  Demux2/2 -> Bus Creator/8  "dy"
  Integrator2/1 -> Demux3/1, MATLAB Function2/2(pqr), MATLAB Function1/1(pqr), MATLAB Function3/1(pqr)
  THRUST/1 -> MATLAB Function2/4(F)
  MOMENT/1 -> MATLAB Function3/2(M)

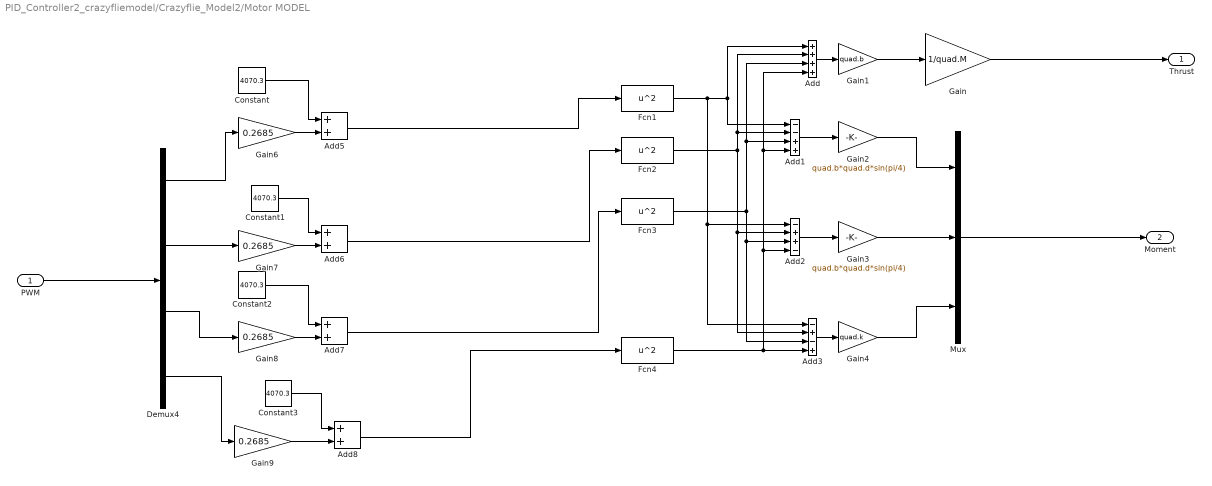
== system PID_Controller2_crazyfliemodel/Crazyflie_Model2/Motor MODEL ==
  PWM : Inport
  Add : Sum  Inputs=++++
  Add1 : Sum  Inputs=--++
  Add2 : Sum  Inputs=-++-
  Add3 : Sum  Inputs=-+-+
  Add{5..8} (4 alike) : Sum
  Constant{,1..3} (4 alike) : Constant  Value=4070.3
  Demux4 : Demux
  Fcn{1..4} (4 alike) : Fcn  Expr=u^2
  Gain : Gain  Gain=1/quad.M
  Gain1 : Gain  Gain=quad.b
  Gain2 : Gain  Gain=quad.b*quad.d*sin(pi/4)
  Gain3 : Gain  Gain=quad.b*quad.d*sin(pi/4)
  Gain4 : Gain  Gain=quad.k
  Gain{6..9} (4 alike) : Gain  Gain=0.2685
  Mux : Mux  Inputs=3
  Thrust : Outport
  Moment : Outport  Port=2
  wires:
  Fcn1/1 -> Add/1, Add1/1, Add2/1, Add3/1
  Add1/1 -> Gain2/1
  Add6/1 -> Fcn2/1
  Fcn3/1 -> Add1/3, Add/3, Add2/3, Add3/3
  Add/1 -> Gain1/1
  Gain2/1 -> Mux/1
  Gain4/1 -> Mux/3
  Fcn2/1 -> Add2/2, Add3/2, Add1/2, Add/2
  Add3/1 -> Gain4/1
  Add2/1 -> Gain3/1
  Add7/1 -> Fcn3/1
  Mux/1 -> Moment/1
  Gain1/1 -> Gain/1
  Add5/1 -> Fcn1/1
  Gain3/1 -> Mux/2
  Add8/1 -> Fcn4/1
  Fcn4/1 -> Add/4, Add1/4, Add2/4, Add3/4
  Gain/1 -> Thrust/1
  Constant2/1 -> Add7/1
  PWM/1 -> Demux4/1
  Constant/1 -> Add5/1
  Gain8/1 -> Add7/2
  Demux4/3 -> Gain8/1
  Gain9/1 -> Add8/2
  Constant1/1 -> Add6/1
  Demux4/2 -> Gain7/1
  Demux4/1 -> Gain6/1
  Constant3/1 -> Add8/1
  Demux4/4 -> Gain9/1
  Gain7/1 -> Add6/2
  Gain6/1 -> Add5/2

== system PID_Controller2_crazyfliemodel/Controller/Altitude_controller/PID_Altitude ==
  Setpoint : Inport
  Measured : Inport  Port=2
  Derivative : Derivative
  Integrator Limited : Integrator  LimitOutput=on  UpperSaturationLimit=1000  LowerSaturationLimit=-1000
  Kd : Gain  Gain=9000  OutMin=[-200]  OutMax=[200]
  Ki : Gain  Gain=3500  OutMin=[-200]  OutMax=[200]
  Kp : Gain  Gain=11000  OutMin=[-200]  OutMax=[200]
  Sum5 : Sum  Inputs=+++
  Sum6 : Sum  Inputs=+-|
  Adjust : Outport
  wires:
  Derivative/1 -> Kd/1
  Integrator Limited/1 -> Ki/1
  Sum6/1 -> Kp/1, Integrator Limited/1, Derivative/1  "pid_error"
  Kd/1 -> Sum5/3
  Kp/1 -> Sum5/1
  Ki/1 -> Sum5/2
  Setpoint/1 -> Sum6/1  "pid_desired"
  Measured/1 -> Sum6/2  "measured"
  Sum5/1 -> Adjust/1

== system PID_Controller2_crazyfliemodel/Controller/Attitude_controller/PID_pitch_Rate2 ==
  Setpoint : Inport
  Measured : Inport  Port=2
  Derivative : Derivative
  Integrator Limited : Integrator  LimitOutput=on  UpperSaturationLimit=20  LowerSaturationLimit=-20
  Kd : Gain  Gain=0  OutMin=[-200]  OutMax=[200]
  Ki : Gain  Gain=2  OutMin=[-200]  OutMax=[200]
  Kp : Gain  Gain=3.5  OutMin=[-200]  OutMax=[200]
  Scope : Scope
  Sum5 : Sum  Inputs=+++
  Sum6 : Sum  Inputs=+-|
  Adjust : Outport
  wires:
  Derivative/1 -> Kd/1
  Integrator Limited/1 -> Ki/1, Scope/1
  Sum6/1 -> Kp/1, Integrator Limited/1, Derivative/1  "pid_error"
  Kd/1 -> Sum5/3
  Kp/1 -> Sum5/1
  Sum5/1 -> Adjust/1
  Ki/1 -> Sum5/2
  Setpoint/1 -> Sum6/1  "pid_desired"
  Measured/1 -> Sum6/2  "measured"

== system PID_Controller2_crazyfliemodel/Controller/Attitude_controller/PID_roll_Rate1 ==
  Setpoint : Inport
  Measured : Inport  Port=2
  Derivative : Derivative
  Integrator Limited : Integrator  LimitOutput=on  UpperSaturationLimit=20  LowerSaturationLimit=-20
  Kd : Gain  Gain=0  OutMin=[-200]  OutMax=[200]
  Ki : Gain  Gain=2  OutMin=[-200]  OutMax=[200]
  Kp : Gain  Gain=3.5  OutMin=[-200]  OutMax=[200]
  Scope : Scope
  Sum5 : Sum  Inputs=+++
  Sum6 : Sum  Inputs=+-|
  Adjust : Outport
  wires:
  Measured/1 -> Sum6/2  "measured"
  Setpoint/1 -> Sum6/1  "pid_desired"
  Ki/1 -> Sum5/2
  Sum5/1 -> Adjust/1
  Kp/1 -> Sum5/1
  Kd/1 -> Sum5/3
  Sum6/1 -> Derivative/1, Integrator Limited/1, Kp/1  "pid_error"
  Integrator Limited/1 -> Scope/1, Ki/1
  Derivative/1 -> Kd/1

== system PID_Controller2_crazyfliemodel/Controller/Position_controller/PID_pitch_Rate2 ==
  Setpoint : Inport
  Measured : Inport  Port=2
  Derivative : Derivative
  Integrator Limited : Integrator  LimitOutput=on  UpperSaturationLimit=0.1  LowerSaturationLimit=-0.1
  Kd : Gain  Gain=0  OutMin=[-200]  OutMax=[200]
  Ki : Gain  Gain=2  OutMin=[-200]  OutMax=[200]
  Kp : Gain  Gain=30  OutMin=[-200]  OutMax=[200]
  Scope : Scope
  Sum5 : Sum  Inputs=+++
  Sum6 : Sum  Inputs=+-|
  Adjust : Outport
  wires:
  Measured/1 -> Sum6/2  "measured"
  Setpoint/1 -> Sum6/1  "pid_desired"
  Ki/1 -> Sum5/2
  Sum5/1 -> Adjust/1
  Kp/1 -> Sum5/1
  Kd/1 -> Sum5/3
  Sum6/1 -> Derivative/1, Integrator Limited/1, Kp/1  "pid_error"
  Integrator Limited/1 -> Scope/1, Ki/1
  Derivative/1 -> Kd/1

== system PID_Controller2_crazyfliemodel/Controller/Position_controller/PID_roll_Rate3 ==
  Setpoint : Inport
  Measured : Inport  Port=2
  Derivative : Derivative
  Integrator Limited : Integrator  LimitOutput=on  UpperSaturationLimit=0.1  LowerSaturationLimit=-0.1
  Kd : Gain  Gain=0  OutMin=[-200]  OutMax=[200]
  Ki : Gain  Gain=-2  OutMin=[-200]  OutMax=[200]
  Kp : Gain  Gain=-30  OutMin=[-200]  OutMax=[200]
  Scope : Scope
  Sum5 : Sum  Inputs=+++
  Sum6 : Sum  Inputs=+-|
  Adjust : Outport
  wires:
  Derivative/1 -> Kd/1
  Integrator Limited/1 -> Ki/1, Scope/1
  Sum6/1 -> Kp/1, Integrator Limited/1, Derivative/1  "pid_error"
  Kd/1 -> Sum5/3
  Kp/1 -> Sum5/1
  Sum5/1 -> Adjust/1
  Ki/1 -> Sum5/2
  Setpoint/1 -> Sum6/1  "pid_desired"
  Measured/1 -> Sum6/2  "measured"

== system PID_Controller2_crazyfliemodel/Controller/Rate_controller/PID_Roll_Rate1 ==
  Setpoint : Inport
  Measured : Inport  Port=2
  Derivative : Derivative
  Integrator Limited : Integrator  LimitOutput=on  UpperSaturationLimit=1000  LowerSaturationLimit=-1000
  Kd : Gain  Gain=0  OutMin=[-200]  OutMax=[200]
  Ki : Gain  Gain=0  OutMin=[-200]  OutMax=[200]
  Kp : Gain  Gain=70  OutMin=[-200]  OutMax=[200]
  Sum5 : Sum  Inputs=+++
  Sum6 : Sum  Inputs=+-|
  Adjust : Outport
  wires:
  Measured/1 -> Sum6/2  "measured"
  Setpoint/1 -> Sum6/1  "pid_desired"
  Ki/1 -> Sum5/2
  Sum5/1 -> Adjust/1
  Kp/1 -> Sum5/1
  Kd/1 -> Sum5/3
  Sum6/1 -> Derivative/1, Integrator Limited/1, Kp/1  "pid_error"
  Integrator Limited/1 -> Ki/1
  Derivative/1 -> Kd/1

== system PID_Controller2_crazyfliemodel/Controller/Rate_controller/PID_Roll_Rate3 ==
  Setpoint : Inport
  Measured : Inport  Port=2
  Derivative : Derivative
  Integrator Limited : Integrator  LimitOutput=on  UpperSaturationLimit=1000  LowerSaturationLimit=-1000
  Kd : Gain  Gain=0  OutMin=[-200]  OutMax=[200]
  Ki : Gain  Gain=0  OutMin=[-200]  OutMax=[200]
  Kp : Gain  Gain=70  OutMin=[-200]  OutMax=[200]
  Scope : Scope
  Sum5 : Sum  Inputs=+++
  Sum6 : Sum  Inputs=+-|
  Adjust : Outport
  wires:
  Derivative/1 -> Kd/1
  Integrator Limited/1 -> Ki/1, Scope/1
  Sum6/1 -> Kp/1, Integrator Limited/1, Derivative/1  "pid_error"
  Kd/1 -> Sum5/3
  Kp/1 -> Sum5/1
  Sum5/1 -> Adjust/1
  Ki/1 -> Sum5/2
  Setpoint/1 -> Sum6/1  "pid_desired"
  Measured/1 -> Sum6/2  "measured"

== system PID_Controller2_crazyfliemodel/Controller/Rate_controller/PID_YAW_Rate1 ==
  Setpoint : Inport
  Measured : Inport  Port=2
  Derivative : Derivative
  Integrator Limited : Integrator  LimitOutput=on  UpperSaturationLimit=1000  LowerSaturationLimit=-1000
  Kd : Gain  Gain=0  OutMin=[-200]  OutMax=[200]
  Ki : Gain  Gain=16.7  OutMin=[-200]  OutMax=[200]
  Kp : Gain  Gain=70  OutMin=[-200]  OutMax=[200]
  Scope : Scope
  Sum5 : Sum  Inputs=+++
  Sum6 : Sum  Inputs=+-|
  Adjust : Outport
  wires:
  Measured/1 -> Sum6/2  "measured"
  Setpoint/1 -> Sum6/1  "pid_desired"
  Ki/1 -> Sum5/2
  Sum5/1 -> Adjust/1
  Kp/1 -> Sum5/1
  Kd/1 -> Sum5/3
  Sum6/1 -> Derivative/1, Integrator Limited/1, Kp/1  "pid_error"
  Integrator Limited/1 -> Scope/1, Ki/1
  Derivative/1 -> Kd/1

== system PID_Controller2_crazyfliemodel/Controller1/Altitude_controller/PID_Altitude ==
  Setpoint : Inport
  Measured : Inport  Port=2
  Derivative : Derivative
  Integrator Limited : Integrator  LimitOutput=on  UpperSaturationLimit=1000  LowerSaturationLimit=-1000
  Kd : Gain  Gain=9000  OutMin=[-200]  OutMax=[200]
  Ki : Gain  Gain=3500  OutMin=[-200]  OutMax=[200]
  Kp : Gain  Gain=11000  OutMin=[-200]  OutMax=[200]
  Sum5 : Sum  Inputs=+++
  Sum6 : Sum  Inputs=+-|
  Adjust : Outport
  wires:
  Derivative/1 -> Kd/1
  Integrator Limited/1 -> Ki/1
  Sum6/1 -> Kp/1, Integrator Limited/1, Derivative/1  "pid_error"
  Kd/1 -> Sum5/3
  Kp/1 -> Sum5/1
  Ki/1 -> Sum5/2
  Setpoint/1 -> Sum6/1  "pid_desired"
  Measured/1 -> Sum6/2  "measured"
  Sum5/1 -> Adjust/1

== system PID_Controller2_crazyfliemodel/Controller1/Attitude_controller/PID_Roll_Rate1 ==
  Setpoint : Inport
  Measured : Inport  Port=2
  Derivative : Derivative
  Integrator Limited : Integrator  LimitOutput=on  UpperSaturationLimit=20  LowerSaturationLimit=-20
  Kd : Gain  Gain=0  OutMin=[-200]  OutMax=[200]
  Ki : Gain  Gain=2  OutMin=[-200]  OutMax=[200]
  Kp : Gain  Gain=3.5  OutMin=[-200]  OutMax=[200]
  Scope : Scope
  Sum5 : Sum  Inputs=+++
  Sum6 : Sum  Inputs=+-|
  Adjust : Outport
  wires:
  Measured/1 -> Sum6/2  "measured"
  Setpoint/1 -> Sum6/1  "pid_desired"
  Ki/1 -> Sum5/2
  Sum5/1 -> Adjust/1
  Kp/1 -> Sum5/1
  Kd/1 -> Sum5/3
  Sum6/1 -> Derivative/1, Integrator Limited/1, Kp/1  "pid_error"
  Integrator Limited/1 -> Scope/1, Ki/1
  Derivative/1 -> Kd/1

== system PID_Controller2_crazyfliemodel/Controller1/Attitude_controller/PID_Roll_Rate2 ==
  Setpoint : Inport
  Measured : Inport  Port=2
  Derivative : Derivative
  Integrator Limited : Integrator  LimitOutput=on  UpperSaturationLimit=20  LowerSaturationLimit=-20
  Kd : Gain  Gain=0  OutMin=[-200]  OutMax=[200]
  Ki : Gain  Gain=2  OutMin=[-200]  OutMax=[200]
  Kp : Gain  Gain=3.5  OutMin=[-200]  OutMax=[200]
  Scope : Scope
  Sum5 : Sum  Inputs=+++
  Sum6 : Sum  Inputs=+-|
  Adjust : Outport
  wires:
  Derivative/1 -> Kd/1
  Integrator Limited/1 -> Ki/1, Scope/1
  Sum6/1 -> Kp/1, Integrator Limited/1, Derivative/1  "pid_error"
  Kd/1 -> Sum5/3
  Kp/1 -> Sum5/1
  Sum5/1 -> Adjust/1
  Ki/1 -> Sum5/2
  Setpoint/1 -> Sum6/1  "pid_desired"
  Measured/1 -> Sum6/2  "measured"

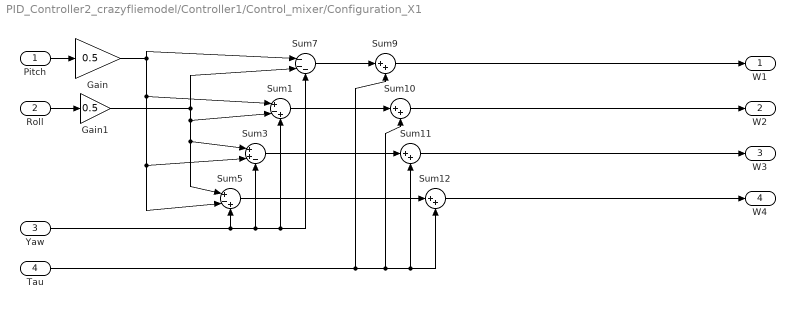
== system PID_Controller2_crazyfliemodel/Controller1/Control_mixer/Configuration_X1 ==
  Pitch : Inport
  Roll : Inport  Port=2
  Yaw : Inport  Port=3
  Tau : Inport  Port=4
  Gain : Gain  Gain=0.5
  Gain1 : Gain  Gain=0.5
  Sum1 : Sum  Inputs=|+-+  SaturateOnIntegerOverflow=on  InputSameDT=on  OutDataTypeStr=Inherit: Same as first input
  Sum{9..12} (4 alike) : Sum  Inputs=|++  SaturateOnIntegerOverflow=on  InputSameDT=on  OutDataTypeStr=Inherit: Same as first input
  Sum3 : Sum  Inputs=|++-  SaturateOnIntegerOverflow=on  InputSameDT=on  OutDataTypeStr=Inherit: Same as first input
  Sum5 : Sum  Inputs=|+-+  SaturateOnIntegerOverflow=on  InputSameDT=on  OutDataTypeStr=Inherit: Same as first input
  Sum7 : Sum  Inputs=|---  SaturateOnIntegerOverflow=on  InputSameDT=on  OutDataTypeStr=Inherit: Same as first input
  W1 : Outport
  W2 : Outport  Port=2
  W3 : Outport  Port=3
  W4 : Outport  Port=4
  wires:
  Sum3/1 -> Sum11/1
  Yaw/1 -> Sum5/3, Sum3/3, Sum7/3, Sum1/3
  Tau/1 -> Sum11/2, Sum12/2, Sum10/2, Sum9/2
  Sum5/1 -> Sum12/1
  Sum7/1 -> Sum9/1
  Sum1/1 -> Sum10/1
  Roll/1 -> Gain1/1
  Pitch/1 -> Gain/1
  Gain/1 -> Sum7/1, Sum1/1, Sum5/2, Sum3/2
  Gain1/1 -> Sum7/2, Sum1/2, Sum5/1, Sum3/1
  Sum9/1 -> W1/1
  Sum10/1 -> W2/1
  Sum11/1 -> W3/1
  Sum12/1 -> W4/1

== system PID_Controller2_crazyfliemodel/Controller1/Position_controller/PID_Roll_Rate2 ==
  Setpoint : Inport
  Measured : Inport  Port=2
  Derivative : Derivative
  Integrator Limited : Integrator  LimitOutput=on  UpperSaturationLimit=0.1  LowerSaturationLimit=-0.1
  Kd : Gain  Gain=0  OutMin=[-200]  OutMax=[200]
  Ki : Gain  Gain=2  OutMin=[-200]  OutMax=[200]
  Kp : Gain  Gain=30  OutMin=[-200]  OutMax=[200]
  Scope : Scope
  Sum5 : Sum  Inputs=+++
  Sum6 : Sum  Inputs=+-|
  Adjust : Outport
  wires:
  Measured/1 -> Sum6/2  "measured"
  Setpoint/1 -> Sum6/1  "pid_desired"
  Ki/1 -> Sum5/2
  Sum5/1 -> Adjust/1
  Kp/1 -> Sum5/1
  Kd/1 -> Sum5/3
  Sum6/1 -> Derivative/1, Integrator Limited/1, Kp/1  "pid_error"
  Integrator Limited/1 -> Scope/1, Ki/1
  Derivative/1 -> Kd/1

== system PID_Controller2_crazyfliemodel/Controller1/Position_controller/PID_Roll_Rate3 ==
  Setpoint : Inport
  Measured : Inport  Port=2
  Derivative : Derivative
  Integrator Limited : Integrator  LimitOutput=on  UpperSaturationLimit=0.1  LowerSaturationLimit=-0.1
  Kd : Gain  Gain=0  OutMin=[-200]  OutMax=[200]
  Ki : Gain  Gain=-2  OutMin=[-200]  OutMax=[200]
  Kp : Gain  Gain=-30  OutMin=[-200]  OutMax=[200]
  Scope : Scope
  Sum5 : Sum  Inputs=+++
  Sum6 : Sum  Inputs=+-|
  Adjust : Outport
  wires:
  Derivative/1 -> Kd/1
  Integrator Limited/1 -> Ki/1, Scope/1
  Sum6/1 -> Kp/1, Integrator Limited/1, Derivative/1  "pid_error"
  Kd/1 -> Sum5/3
  Kp/1 -> Sum5/1
  Sum5/1 -> Adjust/1
  Ki/1 -> Sum5/2
  Setpoint/1 -> Sum6/1  "pid_desired"
  Measured/1 -> Sum6/2  "measured"
